simulink model "master_slave"  (R2020a)
settings: Solver=VariableStepAuto  StartTime=0.0  StopTime=7  RelTol=1e-3
values from neighbouring files (symbols this model uses):
  Be = 5    [Teleop_parameters.m]
  Bh = 0.02    [Teleop_parameters.m]
  Fc_h = 5    [Teleop_parameters.m]
  Jh = 0.02    [Teleop_parameters.m]
  k_m = 19.34    [Teleop_parameters.m]
  Kc2v_m = 2    [Teleop_parameters.m]
  Kc2v_s = 2    [Teleop_parameters.m]
  Kd_h = 0.5    [Teleop_parameters.m]
  Kd_m = 0.005    [Teleop_parameters.m]
  Kd_s = 0.5    [Teleop_parameters.m]
  Ke = 10    [Teleop_parameters.m]
  Kp_h = 1.2    [Teleop_parameters.m]
  Kp_m = 0.01    [Teleop_parameters.m]
  Kp_s = 1    [Teleop_parameters.m]
  Kt2c_m = 1.182    [Teleop_parameters.m]
  Kt2c_s = 1.182    [Teleop_parameters.m]
  lArm_m = 0.1    [Teleop_parameters.m]
  lArm_s = 0.1    [Teleop_parameters.m]
  maxCurrent_m = 4.5    [Teleop_parameters.m]
  maxCurrent_s = 4.5    [Teleop_parameters.m]
  qe = 0.5    [Teleop_parameters.m]
  tau_m = 1.217    [Teleop_parameters.m]
settings Model: Creator=kriato  LastModifiedBy=giova

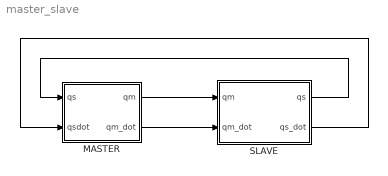
== system master_slave ==
  MASTER : Subsystem
  SLAVE : Subsystem
  wires:
  SLAVE/1(qs) -> MASTER/1("qs ")
  SLAVE/2(qs_dot) -> MASTER/2(qsdot)
  MASTER/1(qm) -> SLAVE/1(qm)
  MASTER/2(qm_dot) -> SLAVE/2(qm_dot)

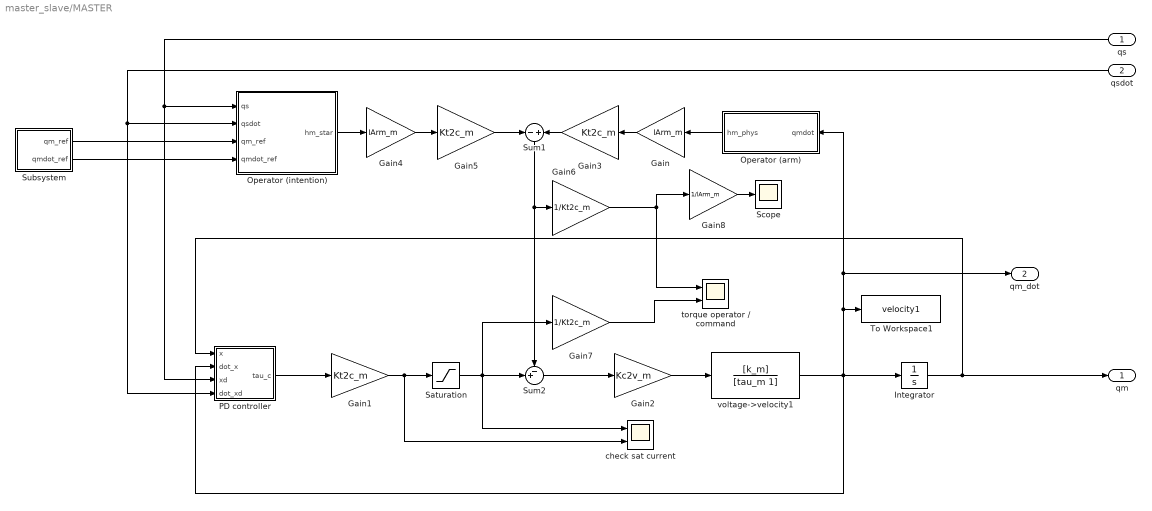
== system master_slave/MASTER ==
  "qs " : Inport
  qsdot : Inport  Port=2
  Gain : Gain  Gain=lArm_m
  Gain1 : Gain  Gain=Kt2c_m
  Gain2 : Gain  Gain=Kc2v_m
  Gain3 : Gain  Gain=Kt2c_m
  Gain4 : Gain  Gain=lArm_m
  Gain5 : Gain  Gain=Kt2c_m
  Gain6 : Gain  Gain=1/Kt2c_m
  Gain7 : Gain  Gain=1/Kt2c_m
  Gain8 : Gain  Gain=1/lArm_m
  Integrator : Integrator
  Operator (arm) : Subsystem
  Operator (intention) : Subsystem
  PD controller : Subsystem
  Saturation : Saturate  UpperLimit=maxCurrent_m  LowerLimit=-maxCurrent_m
  Scope : Scope
  Subsystem : Subsystem
  Sum1 : Sum  Inputs=-+
  Sum2 : Sum  Inputs=-+|
  To Workspace1 : ToWorkspace  VariableName=velocity1  SaveFormat=Timeseries  SampleTime=-1
  check sat current : Scope  NumInputPorts=2
  torque operator / command : Scope  NumInputPorts=2
  voltage->velocity1 : TransferFcn  Numerator=[k_m]  Denominator=[tau_m 1]
  qm : Outport
  qm_dot : Outport  Port=2
  wires:
  Gain7/1 -> torque operator / command/2
  Operator (intention)/1(hm_star) -> Gain4/1
  Subsystem/2(qmdot_ref) -> Operator (intention)/4(qmdot_ref)
  Gain3/1 -> Sum1/2
  Operator (arm)/1(hm_phys) -> Gain/1
  Integrator/1 -> qm/1, PD controller/1(x)
  "qs "/1 -> PD controller/3(xd), Operator (intention)/1(qs)
  qsdot/1 -> PD controller/4(dot_xd), Operator (intention)/2(qsdot)
  Gain4/1 -> Gain5/1
  Gain2/1 -> voltage->velocity1/1
  Subsystem/1(qm_ref) -> Operator (intention)/3(qm_ref)
  Gain/1 -> Gain3/1
  Gain6/1 -> torque operator / command/1, Gain8/1
  voltage->velocity1/1 -> Operator (arm)/1(qmdot), qm_dot/1, To Workspace1/1, PD controller/2(dot_x), Integrator/1
  Gain5/1 -> Sum1/1
  Saturation/1 -> Gain7/1, Sum2/2, check sat current/1
  PD controller/1(tau_c) -> Gain1/1
  Sum1/1 -> Sum2/1, Gain6/1
  Sum2/1 -> Gain2/1
  Gain1/1 -> check sat current/2, Saturation/1
  Gain8/1 -> Scope/1

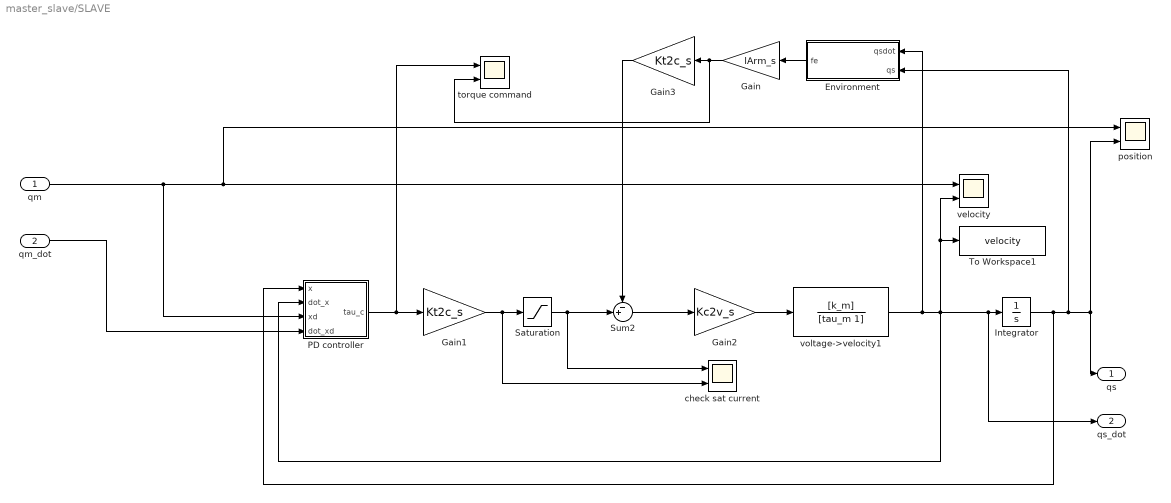
== system master_slave/SLAVE ==
  qm : Inport
  qm_dot : Inport  Port=2
  Environment : Subsystem
  Gain : Gain  Gain=lArm_s
  Gain1 : Gain  Gain=Kt2c_s
  Gain2 : Gain  Gain=Kc2v_s
  Gain3 : Gain  Gain=Kt2c_s
  Integrator : Integrator
  PD controller : Subsystem
  Saturation : Saturate  UpperLimit=maxCurrent_s  LowerLimit=-maxCurrent_s
  Sum2 : Sum  Inputs=-+|
  To Workspace1 : ToWorkspace  VariableName=velocity  SaveFormat=Timeseries  SampleTime=-1
  check sat current : Scope  NumInputPorts=2
  position : Scope  NumInputPorts=2
  torque command : Scope  NumInputPorts=2
  velocity : Scope  NumInputPorts=2
  voltage->velocity1 : TransferFcn  Numerator=[k_m]  Denominator=[tau_m 1]
  qs : Outport
  qs_dot : Outport  Port=2
  wires:
  Integrator/1 -> PD controller/1(x), qs/1, position/2, Environment/2(qs)
  Gain/1 -> torque command/2, Gain3/1
  PD controller/1(tau_c) -> torque command/1, Gain1/1
  qm/1 -> PD controller/3(xd), velocity/1, position/1
  Gain1/1 -> check sat current/2, Saturation/1
  Saturation/1 -> Sum2/2, check sat current/1
  Sum2/1 -> Gain2/1
  Environment/1(fe) -> Gain/1
  Gain3/1 -> Sum2/1
  Gain2/1 -> voltage->velocity1/1
  voltage->velocity1/1 -> Environment/1(qsdot), velocity/2, To Workspace1/1, PD controller/2(dot_x), qs_dot/1, Integrator/1
  qm_dot/1 -> PD controller/4(dot_xd)

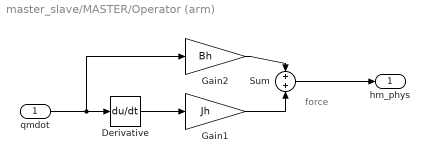
== system master_slave/MASTER/Operator (arm) ==
  note: force
  qmdot : Inport
  Derivative : Derivative  CoefficientInTFapproximation=0.001
  Gain1 : Gain  Gain=Jh
  Gain2 : Gain  Gain=Bh
  Sum : Sum  Inputs=+|+
  hm_phys : Outport  VectorParamsAs1DForOutWhenUnconnected=off
  wires:
  qmdot/1 -> Gain2/1, Derivative/1
  Sum/1 -> hm_phys/1
  Derivative/1 -> Gain1/1
  Gain2/1 -> Sum/1
  Gain1/1 -> Sum/2

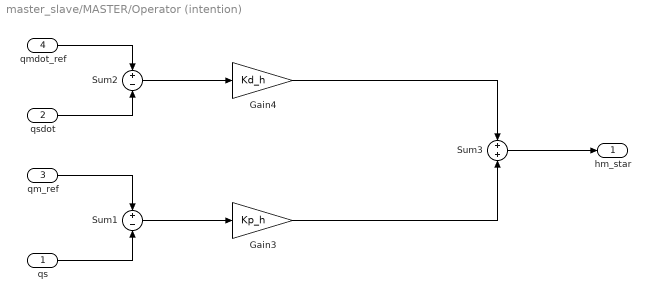
== system master_slave/MASTER/Operator (intention) ==
  qs : Inport
  qsdot : Inport  Port=2
  qm_ref : Inport  Port=3
  qmdot_ref : Inport  Port=4
  Gain3 : Gain  Gain=Kp_h
  Gain4 : Gain  Gain=Kd_h
  Sum1 : Sum  Inputs=+|-
  Sum2 : Sum  Inputs=+|-
  Sum3 : Sum  Inputs=+|+
  hm_star : Outport  VectorParamsAs1DForOutWhenUnconnected=off
  wires:
  qs/1 -> Sum1/2
  qm_ref/1 -> Sum1/1
  qmdot_ref/1 -> Sum2/1
  Sum1/1 -> Gain3/1
  qsdot/1 -> Sum2/2
  Sum2/1 -> Gain4/1
  Gain4/1 -> Sum3/1
  Gain3/1 -> Sum3/2
  Sum3/1 -> hm_star/1

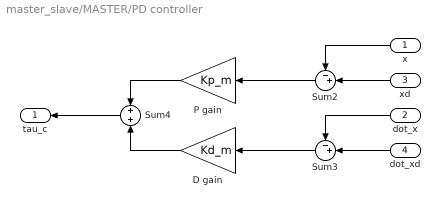
== system master_slave/MASTER/PD controller ==
  x : Inport
  dot_x : Inport  Port=2
  xd : Inport  Port=3
  dot_xd : Inport  Port=4
  D gain : Gain  Gain=Kd_m
  P gain : Gain  Gain=Kp_m
  Sum2 : Sum  Inputs=-+|
  Sum3 : Sum  Inputs=-+|
  Sum4 : Sum
  tau_c : Outport  VectorParamsAs1DForOutWhenUnconnected=off
  wires:
  D gain/1 -> Sum4/2
  dot_x/1 -> Sum3/1
  dot_xd/1 -> Sum3/2
  x/1 -> Sum2/1
  xd/1 -> Sum2/2
  Sum3/1 -> D gain/1
  P gain/1 -> Sum4/1
  Sum4/1 -> tau_c/1
  Sum2/1 -> P gain/1

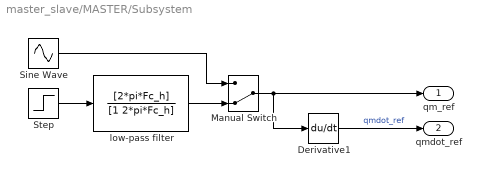
== system master_slave/MASTER/Subsystem ==
  Derivative1 : Derivative  CoefficientInTFapproximation=0.001
  Manual Switch : ManualSwitch  CurrentSetting=0
  Sine Wave : Sin  SampleTime=0
  Step : Step  SampleTime=0
  low-pass filter : TransferFcn  Numerator=[2*pi*Fc_h]  Denominator=[1 2*pi*Fc_h]
  qm_ref : Outport
  qmdot_ref : Outport  Port=2
  wires:
  low-pass filter/1 -> Manual Switch/2
  Manual Switch/1 -> qm_ref/1, Derivative1/1
  Derivative1/1 -> qmdot_ref/1  "qmdot_ref"
  Step/1 -> low-pass filter/1
  Sine Wave/1 -> Manual Switch/1

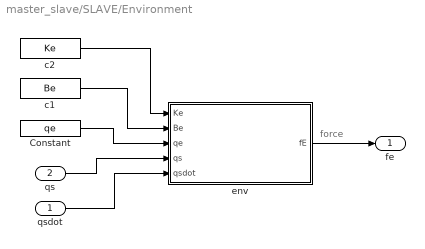
== system master_slave/SLAVE/Environment ==
  note: force
  qsdot : Inport
  qs : Inport  Port=2
  Constant : Constant  Value=qe  SampleTime=0
  c1 : Constant  Value=Be  SampleTime=0
  c2 : Constant  Value=Ke  SampleTime=0
  env : MATLAB Function  TreatAsAtomicUnit=on
  fe : Outport  VectorParamsAs1DForOutWhenUnconnected=off
  wires:
  Constant/1 -> env/3(qe)
  c1/1 -> env/2(Be)
  c2/1 -> env/1(Ke)
  qs/1 -> env/4(qs)
  qsdot/1 -> env/5(qsdot)
  env/1(fE) -> fe/1

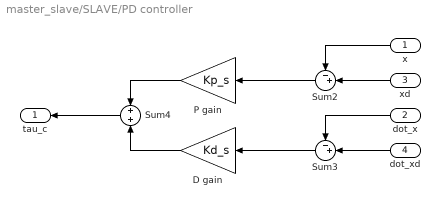
== system master_slave/SLAVE/PD controller ==
  x : Inport
  dot_x : Inport  Port=2
  xd : Inport  Port=3
  dot_xd : Inport  Port=4
  D gain : Gain  Gain=Kd_s
  P gain : Gain  Gain=Kp_s
  Sum2 : Sum  Inputs=-+|
  Sum3 : Sum  Inputs=-+|
  Sum4 : Sum
  tau_c : Outport  VectorParamsAs1DForOutWhenUnconnected=off
  wires:
  D gain/1 -> Sum4/2
  dot_x/1 -> Sum3/1
  dot_xd/1 -> Sum3/2
  x/1 -> Sum2/1
  xd/1 -> Sum2/2
  Sum3/1 -> D gain/1
  P gain/1 -> Sum4/1
  Sum4/1 -> tau_c/1
  Sum2/1 -> P gain/1

== matlab function master_slave/SLAVE/Environment/env ==
  data: Ke input; Be input; qe input; qs input; fE output; qsdot input
function fE  = environment(Ke, Be, qe, qs, qsdot)
if qs > qe
   fE = Ke * (qs - qe) + Be * qsdot;
else
   fE = 0;
end
